simulink model "BoschAEB_Hyd"  (R2021a)
settings: Solver=ode1  StartTime=0.0  StopTime=inf  FixedStep=0.001  RelTol=1e-3
PreLoadFcn:
  | vehicle = 'Car'; if ~length(which('cmself')), cmenv; end
  | BoschAEB_Hyd_bus
InitFcn:
  | vehicle = 'Car'; if ~length(which('cmself')), cmenv; end
  | BoschAEB_Hyd_bus
model workspace (MAT data in the model file):
  CpFront_CpF = 20.55
  CpRear_CpR = 13.93
  Driver_J_Max = 0
  Driver_a_Max = 0
  Normal.Time = [0 0.001 0.002 0.003 0.004 0.005 0.006 0.007 0.008 0.009 0.01 0.011 0.012 0.013 0.014 0.015 0.016 0.017 0.018 0.019 0.02 0.021 0.022 0.023 0.024 0.025 0.026 0.027 0.028 0.029 0.03 0.031 0.032 0.033 0.034 0.035 0.036 0.037 0.038 0.039 0.04 0.041 0.042 0.043 0.044 0.045 0.046 0.047 0.048 0.049 0.05 0.051 0.052 0.053 0.054 0.055 0.056 0.057 0.058 0.059 0.06 0.061 0.062 0.063 0.064 0.065 0.066 0.067 0.068 0.069 0.07 0.071 0.072 0.073 0.074 0.075 0.076 0.077 0.078 0.079 0.08 0.081 0.082 0.083 0.084 0.085 0.086 0.087 0.088 0.089 0.09 0.091 0.092 0.093 0.094 0.095 0.096 0.097 0.098 0.099 0.1 0.101 0.102 0.103 0.104 0.105 0.106 0.107 0.108 0.109 0.11 0.111 0.112 0.113 0.114 0.115 0.116 0.117 0.118 0.119 0.12 0.121 0.122 0.123 0.124 0.125 0.126 0.127 0.128 0.129 0.13 0.131 0.132 0.133 0.134 0.135 0.136 0.137 0.138 0.139 0.14 0.141 0.142 0.143 0.144 0.145 0.146 0.147 0.148 0.149 0.15 0.151 0.152 0.153 0.154 0.155 0.156 0.157 0.158 0.159 0.16 0.161 0.162 0.163 0.164 0.165 0.166 0.167 0.168 0.169 0.17 0.171 0.172 0.173 0.174 0.175 0.176 0.177 0.178 0.179 0.18]
  Normal.PFront = [0 0 0 0 0.00310070886936 0.0234525880553 0.0538384073989 0.0895722138707 0.129687773237 0.173785031088 0.221383232105 0.272222195603 ... (181 elements, 1x181)]
  Normal.PRear = [0 0 0 0 0.0021168217293 0.0160716027731 0.0370648934359 0.0619933799584 0.0902273831398 0.121375511744 0.15487181476 0.190768496749 ... (181 elements, 1x181)]
  PLockFront_PLF = 83
  PLockRear_PLR = 116
  Prefill.Time = [0 0.001 0.002 0.003 0.004 0.005 0.006 0.007 0.008 0.009 0.01 0.011 0.012 0.013 0.014 0.015 0.016 0.017 0.018 0.019 0.02 0.021 0.022 0.023 0.024 0.025 0.026 0.027 0.028 0.029 0.03 0.031 0.032 0.033 0.034 0.035 0.036 0.037 0.038 0.039 0.04 0.041 0.042 0.043 0.044 0.045 0.046 0.047 0.048 0.049 0.05 0.051 0.052 0.053 0.054 0.055 0.056 0.057 0.058 0.059 0.06 0.061 0.062 0.063 0.064 0.065 0.066 0.067 0.068 0.069 0.07 0.071 0.072 0.073 0.074 0.075 0.076 0.077 0.078 0.079 0.08 0.081 0.082 0.083 0.084 0.085 0.086 0.087 0.088 0.089 0.09 0.091 0.092 0.093 0.094 0.095 0.096 0.097 0.098 0.099 0.1 0.101 0.102 0.103 0.104 0.105 0.106 0.107 0.108 0.109 0.11 0.111 0.112 0.113 0.114 0.115 0.116 0.117 0.118 0.119 0.12 0.121 0.122 0.123 0.124 0.125 0.126 0.127 0.128 0.129 0.13 0.131 0.132 0.133 0.134 0.135 0.136 0.137]
  Prefill.PFront = [5.78467898821 6.091319424 6.40107291801 6.71365921309 7.0288309012 7.3463652814 7.66606210222 7.98774089492 8.31123864542 8.63640779326 8.96311451481 9.29123722849 9.65679725976 10.3092987989 10.9605197532 11.7963605271 12.7634878254 13.7269511741 14.6868745531 15.643360084 16.5965019756 17.5463844495 18.4930849842 19.5022539696 20.5352405794 21.5733854213 22.6912303221 23.8043205832 24.9133103613 26.0190561225 27.1220177627 28.2226206799 29.3214348602 30.4189456027 31.5155631169 32.6118476231 33.7081676788 34.8048403761 35.9021411838 37.0003134444 38.0995707865 39.293577279 40.5600980745 41.827936054 43.2593319821 44.6919432032 46.1240959591 47.5563831259 48.9892235287 50.4229159626 51.8580203378 53.2949733663 54.7340264254 56.1757032562 57.6200956508 59.142830666 60.7262500785 62.3332388541 64.0531815525 65.7702023954 67.4842583187 69.1952387894 70.9029723445 72.6072377287 74.3077744949 76.0042902293 77.6964687329 79.3839825708 81.0664998779 82.743686482 84.4152081832 86.080732758 87.7399317152 89.3924818366 91.0380664931 92.676376763 94.307112411 95.9300044136 97.5451424159 99.1525355006 100.75240168 102.344704368 103.929327575 105.506120303 107.074917653 108.635928086 110.190318101 111.737193588 113.276129213 114.806674043 116.328513944 117.841398422 119.417709869 121.035352675 122.71130369 124.425608625 126.123511897 127.807694211 129.47763704 131.133476168 132.775218177 134.402918545 136.016664448 137.61656878 139.202781635 140.775476162 142.334842787 143.881083415 145.414406883 146.935025544 148.443146467 149.938902152 151.422488832 152.894112634 154.353903982 155.802069729 157.238823981 158.664368475 160.078894414 160.826162031 161.4 161.4 161.4 161.4 161.4 161.4 161.4 161.4 161.4 161.4 161.4 161.4 161.4 161.4 161.4 161.4 161.4 161.4]
  Prefill.PRear = [4.04152540895 4.25554846989 4.47191998813 4.69045193024 4.91097879744 5.13335142248 5.35743564978 5.58311055059 5.81026686475 6.03880566087 6.2686371866 6.49967986734 6.73185943537 6.96516097577 7.19962712695 7.43524331311 7.67209047381 7.91020079071 8.14958339978 8.39024267216 8.6321812843 8.87539982515 9.11989752802 9.36567670272 9.61276609097 10.3746350895 11.3038977769 12.3128468675 13.9128844816 15.5007440422 17.0770044164 18.7574808133 20.5635216676 22.3521105927 24.3332518979 26.3381275438 28.320364615 30.2807715298 32.2201064468 34.1390895248 36.0384046497 38.0037628054 40.3131239411 42.5846869204 45.097993662 47.7420702872 50.3338480919 52.8757540124 55.369912942 57.9361854539 60.6575348494 63.3124549456 66.1986248947 69.0391994224 71.7974339036 74.4767088622 77.0811698586 79.6143233776 82.0798076941 84.4813675682 86.8219078967 89.1041115734 91.3304445164 93.5031762893 95.624403395 97.6960643572 99.7199607176 101.697795984 103.631195778 105.521712528 107.370831447 109.17997618 110.950514057 112.683760985 114.380985823 116.043414272 117.672232448 119.328202421 121.00667478 122.718237777 124.421319768 126.070080252 127.669292902 129.223225328 130.735743608 132.212693009 133.664673719 135.089169097 136.48668389 137.857506346 139.20267941 140.523498425 141.821638188 143.101056972 144.364457771 145.615964328 146.865559411 148.125294779 149.38863915 150.653581809 151.917893988 153.179981311 154.438706695 155.69327066 156.943207226 158.188256533 159.428300453 160.663310182 161.893309019 163.118347125 164.338452832 165.553303438 166.762959753 167.96752192 169.166727225 170.360742239 171.549749751 172.733858837 173.913126012 175.356015951 177.017767553 179.132478172 181.504278264 183.953141609 186.504956403 189.135436947 191.825864786 194.587697262 197.403781079 200.21086315 203.030238661 205.868422866 208.727523961 211.493536584 214.244980998 216.984539823 219.70788994 221.457227456]
  Prefill_activation = 1
  WheelRadius_WR = 0.35
libraries: CarMaker4SL x5
Description:
  | CarMaker Plug-in Model Target
settings Model: Creator=MAR3ABT  LastModifiedBy=MAR3ABT
settings RTWCC: Description=CarMaker Plug-in Model Target  SystemTargetFile=CarMaker.tlc  TemplateMakefile=CarMaker_unix-win64.tmf
settings CodeAppCC: MaxIdLength=127
settings STFCustomTargetCC: TargetLangStandard=C99 (ISO)  CombineOutputUpdateFcns=on  CodeInterfacePackaging=Reusable function  GRTInterface=off  GenerateAllocFcn=on  UseToolchainInfoCompliant=off  SystemTargetFile=CarMaker.tlc
settings GRTTargetCC: ParMdlRefBuildCompliant=off  CompOptLevelCompliant=off  ConcurrentExecutionCompliant=off  MatFileLogging=off  CodeInterfacePackaging=Reusable function  CPPClassGenCompliant=off  GenerateAllocFcn=on  UseToolchainInfoCompliant=off  RTWCAPISignals=on  RTWCAPIParams=on

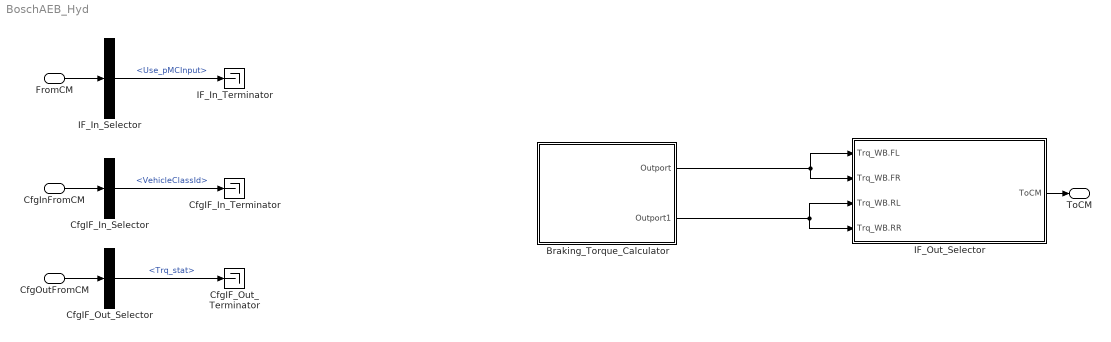
== system BoschAEB_Hyd ==
  FromCM : Inport  OutDataTypeStr=Bus: cmHydBrakeSystemIn
  CfgInFromCM : Inport  Port=2  OutDataTypeStr=Bus: cmHydBrakeSystemCfgIn
  CfgOutFromCM : Inport  Port=3  OutDataTypeStr=Bus: cmHydBrakeSystemCfgOut
  Braking_Torque_Calculator : Subsystem
  CfgIF_In_Selector : BusSelector  OutputSignals=VehicleClassId
  CfgIF_In_Terminator : Terminator
  CfgIF_Out_Selector : BusSelector  OutputSignals=Trq_stat
  CfgIF_Out_Terminator : Terminator
  IF_In_Selector : BusSelector  OutputSignals=Use_pMCInput
  IF_In_Terminator : Terminator
  IF_Out_Selector : Subsystem  mask(Signal Selection){}
      mask help: Signal Selection Block
      settings: OpenFcn=cmSignalSelect('SignalSelection_CB',gcb)
  ToCM : Outport  OutDataTypeStr=Bus: cmHydBrakeSystemOut
  wires:
  FromCM/1 -> IF_In_Selector/1
  IF_In_Selector/1 -> IF_In_Terminator/1  "<Use_pMCInput>"
  IF_Out_Selector/1(ToCM) -> ToCM/1
  CfgInFromCM/1 -> CfgIF_In_Selector/1
  CfgIF_In_Selector/1 -> CfgIF_In_Terminator/1  "<VehicleClassId>"
  CfgOutFromCM/1 -> CfgIF_Out_Selector/1
  CfgIF_Out_Selector/1 -> CfgIF_Out_Terminator/1  "<Trq_stat>"
  Braking_Torque_Calculator/1(Outport) -> IF_Out_Selector/1(Trq_WB.FL), IF_Out_Selector/2(Trq_WB.FR)
  Braking_Torque_Calculator/2(Outport1) -> IF_Out_Selector/3(Trq_WB.RL), IF_Out_Selector/4(Trq_WB.RR)

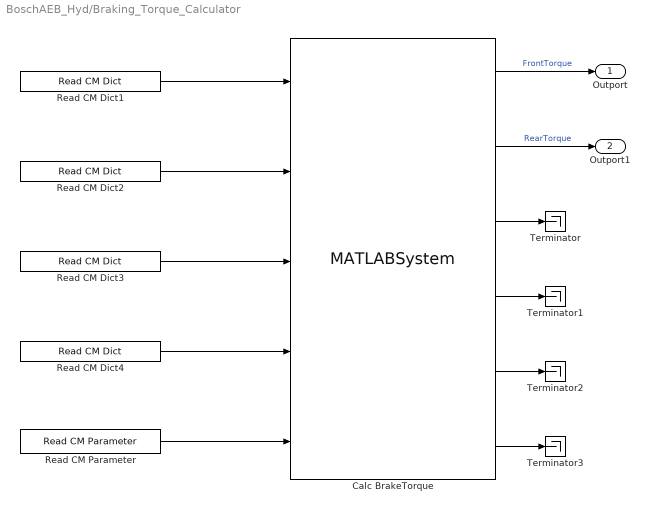
== system BoschAEB_Hyd/Braking_Torque_Calculator ==
  Calc BrakeTorque : MATLABSystem  System=HydrPressureToTrq  Prefill=Prefill_activation  RWheel=WheelRadius_WR  CpFront=CpFront_CpF  CpRear=CpRear_CpR  PLockFront=PLockFront_PLF  PLockRear=PLockRear_PLR  j_Max_Driver=Driver_J_Max  a_Max_Driver=Driver_a_Max  PTime=Normal.Time  PValuesNormal_Front=Normal.PFront  PValuesNormal_Rear=Normal.PRear  PTimePrefill=Prefill.Time  PValuesPrefill_Front=Prefill.PFront  PValuesPrefill_Rear=Prefill.PRear  SimulateUsing=Code generation
      mask Type: HydrPressureToTrq
      mask Display:
      | disp('HydrPressureToTrq');
      | port_label('input',1,'j_Max');
      | port_label('input',2,'a_Start');
      | port_label('input',3,'a_Max');
      | port_label('input',4,'EBA_active');
      | port_label('input',5,'Ego_BodyMass');
      | port_label('output',1,'FrontTorque');
      | port_label('output',2,'RearTorque');
      | port_label('output',3,'pFront');
      | port_label('output',4,'pRear');
      | port_label('output',5,'aEgoTest');
      | port_label('output',6,'aEGO_tgt');
  Read CM Dict1 : CarMaker4SL/Read CM Dict  xname=XCENA5.DACore.j_Max  xsync=off  xstime=Continuous
  Read CM Dict2 : CarMaker4SL/Read CM Dict  xname=XCENA5.DACore.a_Start  xsync=off  xstime=Continuous
  Read CM Dict3 : CarMaker4SL/Read CM Dict  xname=XCENA5.DACore.a_Max  xsync=off  xstime=Continuous
  Read CM Dict4 : CarMaker4SL/Read CM Dict  xname=XCENA5.DACore.EBA_Status  xsync=off  xstime=Continuous
  Read CM Parameter : CarMaker4SL/Read CM Parameter  xfile=Vehicle  xkey=Body.mass  xnout=1  xdefaults=0  xmuxed=on  xstime=Continuous
      settings: SourceProductName=CarMaker4SL
  Terminator{,1..3} (4 alike) : Terminator
  Outport : Outport
  Outport1 : Outport  Port=2
  wires:
  Calc BrakeTorque/2 -> Outport1/1  "RearTorque"
  Calc BrakeTorque/1 -> Outport/1  "FrontTorque"
  Read CM Dict1/1 -> Calc BrakeTorque/1
  Read CM Dict2/1 -> Calc BrakeTorque/2
  Read CM Dict3/1 -> Calc BrakeTorque/3
  Read CM Dict4/1 -> Calc BrakeTorque/4
  Read CM Parameter/1 -> Calc BrakeTorque/5
  Calc BrakeTorque/3 -> Terminator/1
  Calc BrakeTorque/4 -> Terminator1/1
  Calc BrakeTorque/5 -> Terminator2/1
  Calc BrakeTorque/6 -> Terminator3/1

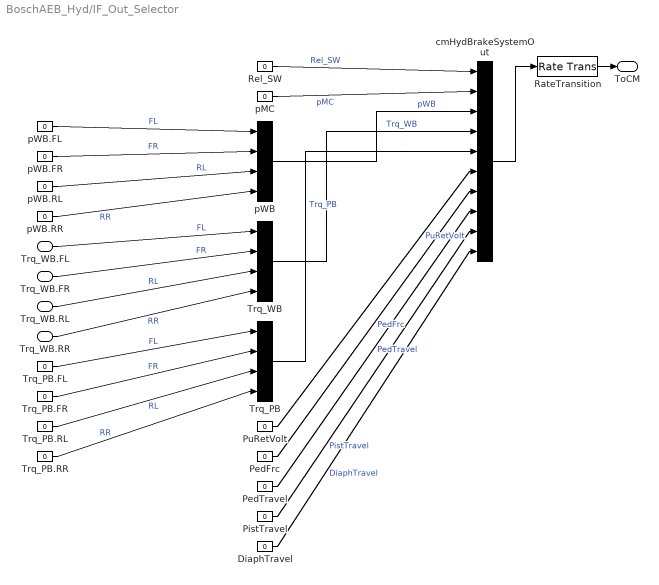
== system BoschAEB_Hyd/IF_Out_Selector ==
  Trq_WB.FL : Inport
  Trq_WB.FR : Inport  Port=2
  Trq_WB.RL : Inport  Port=3
  Trq_WB.RR : Inport  Port=4
  DiaphTravel : Constant  Value=0
  PedFrc : Constant  Value=0
  PedTravel : Constant  Value=0
  PistTravel : Constant  Value=0
  PuRetVolt : Constant  Value=0
  RateTransition : RateTransition  OutPortSampleTime=str2num(get_param(bdroot,'FixedStep'))
  Rel_SW : Constant  Value=0
  Trq_PB : BusCreator  Inputs=4
  Trq_PB.FL : Constant  Value=0
  Trq_PB.FR : Constant  Value=0
  Trq_PB.RL : Constant  Value=0
  Trq_PB.RR : Constant  Value=0
  Trq_WB : BusCreator  Inputs=4
  cmHydBrakeSystemOut : BusCreator  Inputs=10
  pMC : Constant  Value=0
  pWB : BusCreator  Inputs=4
  pWB.FL : Constant  Value=0
  pWB.FR : Constant  Value=0
  pWB.RL : Constant  Value=0
  pWB.RR : Constant  Value=0
  ToCM : Outport
  wires:
  RateTransition/1 -> ToCM/1
  cmHydBrakeSystemOut/1 -> RateTransition/1
  Rel_SW/1 -> cmHydBrakeSystemOut/1  "Rel_SW"
  pMC/1 -> cmHydBrakeSystemOut/2  "pMC"
  pWB/1 -> cmHydBrakeSystemOut/3  "pWB"
  pWB.FL/1 -> pWB/1  "FL"
  pWB.FR/1 -> pWB/2  "FR"
  pWB.RL/1 -> pWB/3  "RL"
  pWB.RR/1 -> pWB/4  "RR"
  Trq_WB/1 -> cmHydBrakeSystemOut/4  "Trq_WB"
  Trq_PB/1 -> cmHydBrakeSystemOut/5  "Trq_PB"
  Trq_PB.FL/1 -> Trq_PB/1  "FL"
  Trq_PB.FR/1 -> Trq_PB/2  "FR"
  Trq_PB.RL/1 -> Trq_PB/3  "RL"
  Trq_PB.RR/1 -> Trq_PB/4  "RR"
  PuRetVolt/1 -> cmHydBrakeSystemOut/6  "PuRetVolt"
  PedFrc/1 -> cmHydBrakeSystemOut/7  "PedFrc"
  PedTravel/1 -> cmHydBrakeSystemOut/8  "PedTravel"
  PistTravel/1 -> cmHydBrakeSystemOut/9  "PistTravel"
  DiaphTravel/1 -> cmHydBrakeSystemOut/10  "DiaphTravel"
  Trq_WB.FL/1 -> Trq_WB/1  "FL"
  Trq_WB.FR/1 -> Trq_WB/2  "FR"
  Trq_WB.RL/1 -> Trq_WB/3  "RL"
  Trq_WB.RR/1 -> Trq_WB/4  "RR"
